simulink model "hdv_hydroelectropowertrain_model"  (R2023b)
settings: Solver=ode1be  StartTime=0.0  StopTime=simulation_length  FixedStep=tsample  MaxStep=tsample
values from neighbouring files (symbols this model uses):
  alpha = 35    [init_model.m]
  Apump = [0 1; 0 0]    [init_model.m]
  available_torque = torque_base+torque_friction_base    [init_model.m]
  Bpump = [0 1]'    [init_model.m]
  btheta_shaft = 2e2    (= 200)    [init_model.m]
  C1 = 10    [init_model.m]
  consumption = [consumption_1, consumption_2, consumption_3, consumption_4,          consumption_5, consumption_6, consumption_7, consumption_8,          consumption_9, consumption_10, consumption_11, consumption_12,          consumption_13, consumption_14, consumption_15, consumption_16          ]    [ic_engine_data.m]
  Cpump = [k 0]    [init_model.m]
  dp_lim = 400    [init_model.m]
  E0 = 3.685    [init_model.m]
  E1 = 0.2156    [init_model.m]
  E2 = 0    [init_model.m]
  E3 = 0    [init_model.m]
  E_1 = -1.031    [init_model.m]
  Elog = -0.05    [init_model.m]
  eta_v_m = 0.98    [init_model.m]
  eta_v_p = 0.97    [init_model.m]
  ki_dp_comp = 1/dp_lim    (= 0.0025)    [init_model.m]
  ki_te_comp = 2/te_lim    [init_model.m]
  kp_ctrl_m = 1    [init_model.m]
  kp_dp_comp = 0.5/dp_lim    (= 0.00125)    [init_model.m]
  kp_te_comp = 1/te_lim    [init_model.m]
  Kpump = acker(Apump,Bpump,poles)    [init_model.m]
  load_blade_enable = 0    [init_model.m]
  Lpump = acker(Apump',Cpump',pole_so)'    [init_model.m]
  M = 125    [init_model.m]
  Ncell = 185    [init_model.m]
  Npump = -1/(Cpump*inv(Apump-Bpump*Kpump)*Bpump)    [init_model.m]
  omega_e_rpm_ref = 1700    [init_model.m]
  omega_l_max_rpm = omega_l_max/(2*pi)*60    (= 50.3075969543)    [init_model.m]
  q1Kalman = tsample^2*1e-2    (= 1e-08)    [init_model.m]
  q2Kalman = tsample^1*1e-1    (= 0.0001)    [init_model.m]
  q3Kalman = 0    [init_model.m]
  Qhr = 400    [init_model.m]
  R0 = 0.015    [init_model.m]
  R1 = 0.015    [init_model.m]
  R_tg = 1.16/2    (= 0.58)    [init_model.m]
  rKalman = 1    [init_model.m]
  rpm_base = [620 700 800 900 1000 1100 1200 1300 1400 1500 1600 1700 1800      1900 2000 2100]    [ic_engine_data.m]
  rpm_consumption = rpm_base    [ic_engine_data.m]
  simulation_length = 245    [init_model.m]
  tau_load = 75e3    (= 75000)    [init_model.m]
  tau_load_max = 1600*41.4    (= 66240)    [init_model.m]
  Tc = tsample    (= 0.001)    [init_model.m]
  torque_base = [max(torque_16_data) max(torque_15_data) max(torque_14_data)      max(torque_13_data) max(torque_12_data) max(torque_11_data)      max(torque_10_data) max(torque_9_data) max(torque_8_data)      max(torque_7_data) max(torque_6_data) max(torque_5_data)      max(torque_4_data) max(torque_3_data) max(torque_2_data)      max(torque_1_data)]    [ic_engine_data.m]
  torque_consumption = torque_reference    [ic_engine_data.m]
  torque_friction_base = -(rpm_base./60*2*pi)*0.25-(rpm_base./60*2*pi).^2*5.2e-4    [ic_engine_data.m]
  tsample = 1e-3    (= 0.001)    [init_model.m]
  v_track1_ref = 8    [init_model.m]
  v_track2_ref = 8    [init_model.m]
  valve_mmorifice_max = 2.75    [init_model.m]
  xv_m_max = 1.2    [init_model.m]
undefined symbols (not defined in the file or in its folder): magnitude
libraries: fl_lib x381, nesl_utility x162, linear_swashplate_ctrl_lib x8, flexshaft_lib x5, bichamber_piston_lib x5, variable_displacement_motor_lib x4, variable_displacement_pump_lib x4, fixed_displacement_pump_lib x4, relief_valve_lib x4, inverse_shuttle_valve_lib x4, hydrostatic_threeway_valve_bichamber_piston_lib x4, hydrostatic_fourway_valve_bichamber_piston_lib x4
(part 1 of 9)
settings Model: SimulationMode=accelerator  Creator=dbagn  LastModifiedBy=dbagn
settings SolverCC: NumberNewtonIterations=3  AlgebraicLoopSolver=TrustRegion
settings DataIOCC: ReturnWorkspaceOutputs=off
settings DebuggingCC: UnconnectedInputMsg=warning  UnconnectedOutputMsg=warning  UnconnectedLineMsg=warning
settings ModelReferenceCC: EnableRefExpFcnMdlSchedulingChecks=on
settings RTWCC: DLArmComputeVersion=19.05

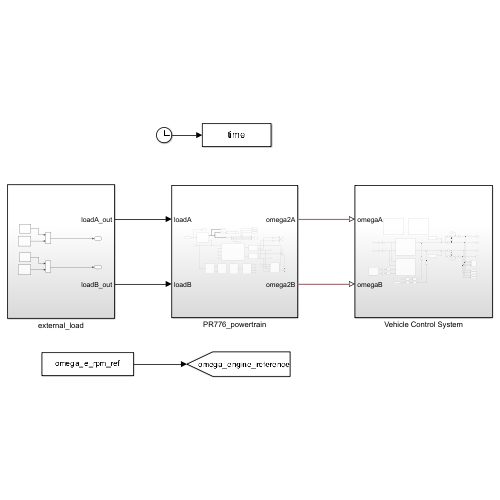
[thumbnail: Simulink's stored preview of the top-level diagram]
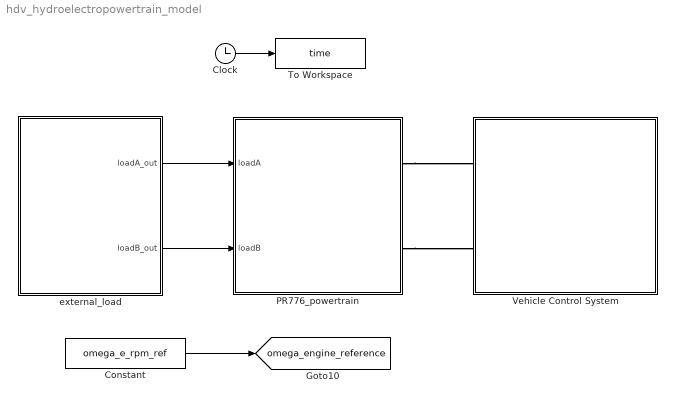
== system hdv_hydroelectropowertrain_model ==
  Clock : Clock
  Constant : Constant  Value=omega_e_rpm_ref
  PR776_powertrain : Subsystem
  To Workspace : ToWorkspace  VariableName=time  SampleTime=Tc
      settings: MaxDataPoints=Nc
  Vehicle Control System : Subsystem
  external_load : Subsystem
  tag scope: omega_engine_reference=global
  wires:
  Clock/1 -> To Workspace/1
  Constant/1 -> [omega_engine_reference]
  external_load/2(loadB_out) -> PR776_powertrain/2(loadB)
  external_load/1(loadA_out) -> PR776_powertrain/1(loadA)
  connections:
  PR776_powertrain/RConn1 -- Vehicle Control System/LConn1
  PR776_powertrain/RConn2 -- Vehicle Control System/LConn2

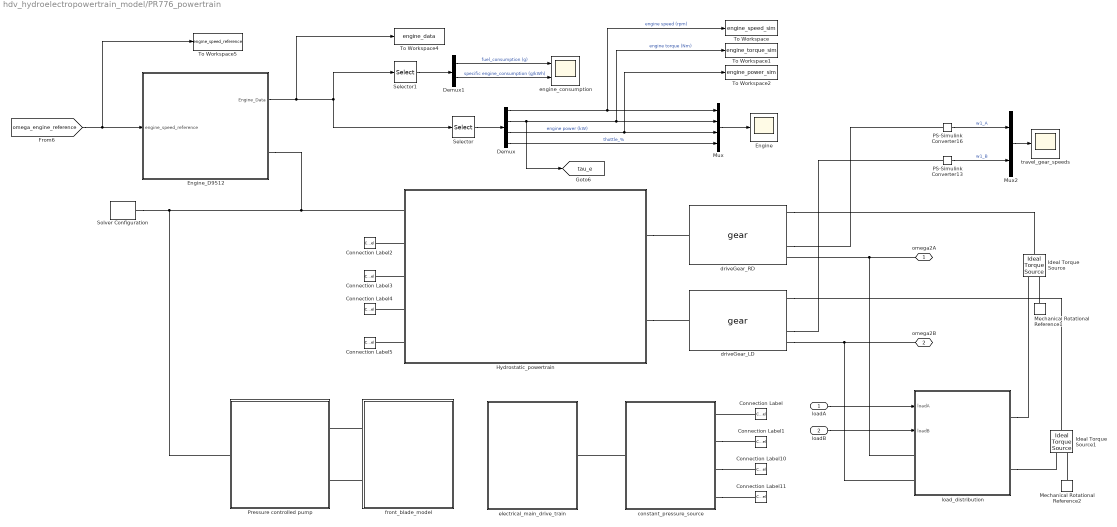
== system hdv_hydroelectropowertrain_model/PR776_powertrain ==
  loadA : Inport
  loadB : Inport  Port=2
  Connection Label : ConnectionLabel  Label=pS1
  Connection Label1 : ConnectionLabel  Label=pT1
  Connection Label10 : ConnectionLabel  Label=pS2
  Connection Label11 : ConnectionLabel  Label=pT2
  Connection Label2 : ConnectionLabel  Label=pS1
  Connection Label3 : ConnectionLabel  Label=pT1
  Connection Label4 : ConnectionLabel  Label=pS2
  Connection Label5 : ConnectionLabel  Label=pT2
  Demux : Demux
  Demux1 : Demux  Outputs=2
  Engine : Scope
  Engine_D9512 : Subsystem  mask(Internal Combustion Engine (ICE)){inertia=7.5, inertia_unit=kg*m^2, init_speed=5, diesel_density=0.85, diesel_density_unit=kg/l, rpm_base=rpm_base, rpm_base_unit=rpm, torque_friction_base=torque_friction_base, torque_friction_base_unit=N*m, torque_base=torque_base, torque_base_unit=N*m, rpm_consumption=rpm_consumption, rpm_consumption_unit=rpm, torque_consumption=torque_consumption, torque_consumption_unit=N*m, consumption=consumption, consumption_unit=g/(kW*hr), kp=2.5e-3, ki=2.5e-2, kd=0}
      mask prompts: init_speed "Initial Speed (RPM)"; diesel_density "Diesel density"; rpm_base "Base Speed Breakpoints"; torque_friction_base "Base Torque Friction Breakpoints"; torque_base "Base Torque Breakpoints"; rpm_consumption "Speed consumption breakpoints"; torque_consumption "Torque consumption breakpoints"; consumption "Consumption map"
      mask help:
      | This component models a generic internal combustion engine, modelled by means of introducing its characteristic performance maps.
      | Maps of main engine performance and of consumption have to be introduced. The component is also provided with a speed controller in which the PID gains can be introduced.
      mask init:
      | engine = [gcb, '/Generic Internal Combustion Engine'];
      | ctrl = [gcb, '/Engine Speed Controller'];
      | 
      | % Engine Parameters
      | set_param([engine],'cshaft_inertia','inertia');
      | set_param([engine],'cshaft_inertia_unit',inertia_unit);
      | set_param([engine],'initial_speed','init_speed');
      | set_param([engine],'diesel_density','diesel_density');
      | set_param([engine],'diesel_density_unit',diesel_density_unit);
      | 
      | % Tables
      | set_param([engine],'rpm_base','rpm_base');
      | set_param([engine],'torque_friction_base', 'torque_friction_base');
      | set_param([engine],'torque_base','torque_base');
      | set_param([engine],'rpm_consumption','rpm_consumption');
      | set_param([engine],'torque_consumption','torque_consumption');
      | set_param([engine],'consumption','consumption');
      | 
      | set_param([engine],'rpm_base_unit',rpm_base_unit);
      | set_param([engine],'torque_friction_base_unit',torque_friction_base_unit);
      | set_param([engine],'torque_base_unit',torque_base_unit);
      | set_param([engine],'rpm_consumption_unit',rpm_consumption_unit);
      | set_param([engine],'torque_consumption_unit',torque_consumption_unit);
      | set_param([engine],'consumption_unit',consumption_unit);
      | 
      | % Speed control
      | set_param([ctrl],'kp','kp');
      | set_param([ctrl],'kint','ki');
      | set_param([ctrl],'kd','kd');
      mask Help: eval('open \documentation\liebherr_engine_D9512_model_description.pdf')
      mask TypeOptions inertia_unit: kg*m^2
      mask TypeOptions diesel_density_unit: kg/l
      mask TypeOptions rpm_base_unit: rpm
      mask TypeOptions torque_friction_base_unit: N*m
      mask TypeOptions torque_base_unit: N*m
      mask TypeOptions rpm_consumption_unit: rpm
      mask TypeOptions torque_consumption_unit: kW
      mask TypeOptions consumption_unit: g/(kW*hr)
      mask DialogControl EngineParameters Prompt: Engine Parameters
      mask DialogControl Container5 Prompt: Engine Main Behaviour
      mask DialogControl Container4 Prompt: Consumption Behaviour
      mask DialogControl ControlParameters Prompt: Control Parameters
      mask Display:
      | modelname = [gcb];
      | % image(imread('Complementary/Pics/ICE.jpg'));
      | 
      | % color('red')
      | % port_label('lconn',1,'wref');
      | color('green')
      | port_label('rconn',1,'D');
      | color('black')
      | port_label('output',1,'Data');
      | port_label('input',1,'Engine Speed Reference');
  Hydrostatic_powertrain : Subsystem
  Ideal Torque Source : fl_lib/Mechanical/Mechanical Sources/Ideal Torque Source
  Ideal Torque Source1 : fl_lib/Mechanical/Mechanical Sources/Ideal Torque Source
  Mechanical Rotational Reference1 : fl_lib/Mechanical/Rotational Elements/Mechanical Rotational Reference
  Mechanical Rotational Reference2 : fl_lib/Mechanical/Rotational Elements/Mechanical Rotational Reference
  Mux : Mux
  Mux2 : Mux  Inputs=2
  PS-Simulink Converter13 : nesl_utility/PS-Simulink Converter  PhysicalDomain=network_engine_domain  SubClassName=ps_output  LeftPortType=input  RightPortType=output  PseudoPeriodic=off  Frequencies=[]  VectorFormat=1-D array  Unit=rpm  AffineConversion=on
  PS-Simulink Converter16 : nesl_utility/PS-Simulink Converter  PhysicalDomain=network_engine_domain  SubClassName=ps_output  LeftPortType=input  RightPortType=output  PseudoPeriodic=off  Frequencies=[]  VectorFormat=1-D array  Unit=rpm  AffineConversion=on
  Pressure controlled pump : Subsystem
  Selector : Selector  InputPortWidth=6  IndexOptions=Index vector (dialog)  Indices=[2 3 1 6]  OutputSizes=1
  Selector1 : Selector  InputPortWidth=6  IndexOptions=Index vector (dialog)  Indices=[5 4]  OutputSizes=1
  Solver Configuration : nesl_utility/Solver Configuration  PhysicalDomain=network_engine_domain  SubClassName=solver  LeftPortType=input  RightPortType=generic  Tones=[]  Harmonics=[]  SimulateNoise=off  Profile=off  UseLocalSampling=off  EnableSwitchedLinearOptims=on  FrequencyDomain=off  UseCCode=off  RelTol=0.001  AbsTol=1e-06  MinStep=1e-09  ToWorkspace=off  RevertToSquareIcSolve=off  NumHomotopyIterations=100  PhasorMode=off  PhasorModeNumHarmonics=1  ConsistencySolver=NEWTON_FTOL  IndexReductionMethod=DerivativeReplacement  DoDC=off  ResidualTolerance=tsample  ConsistencyTolSource=GLOBAL  ConsistencyAbsTol=0.001  ConsistencyRelTol=0.001  ConsistencyTolFactor=0.001  UseLocalSolver=on  LocalSolverChoice=NE_BACKWARD_EULER_ADVANCER  ResolveIndetEquations=on  FunctionEvalNumThread=1  LocalSolverSampleTime=tsample  DoFixedCost=on  MaxNonlinIter=3  MaxModeIter=2  ComputeImpulses=off  ImpulseIterations=2  LinearAlgebra=auto  LinearAlgebraNumThread=0  EquationFormulation=NE_TIME_EF  DelaysMemoryBudget=1024  AutomaticFiltering=on  FilteringTimeConstant=tsample  PartitionStorageMethod=AS_NEEDED  PartitionMemoryBudget=1024  PartitionMethod=ROBUST  MultibodyUseLocalSolver=off  MultibodyLocalSolverChoice=ODE1  MultibodyLocalSolverSampleTime=0.001
  To Workspace : ToWorkspace  VariableName=engine_speed_sim  SampleTime=Tc
      settings: MaxDataPoints=Nc
  To Workspace1 : ToWorkspace  VariableName=engine_torque_sim  SampleTime=Tc
      settings: MaxDataPoints=Nc
  To Workspace2 : ToWorkspace  VariableName=engine_power_sim  SampleTime=Tc
      settings: MaxDataPoints=Nc
  To Workspace4 : ToWorkspace  VariableName=engine_data  SampleTime=Tc
      settings: MaxDataPoints=Nc
  To Workspace5 : ToWorkspace  VariableName=engine_speed_reference  SampleTime=Tc
      settings: MaxDataPoints=Nc
  constant_pressure_source : Subsystem
  driveGear_LD : gear_lib/gear  n1=n_tg  n2=1  b1=b1 %0.02 N*m/(rad/s)  J1=0.25 kg*m^2  b2=track_friction_2 N*m/(rad/s)  J2=2 kg*m^2  k_theta_1=k_theta N*m/rad  w_1_specify=off  w_1_priority=None  w_1=0 rad/s  w_1_nominal_specify=off  w_1_nominal_unit=rad/s  w_1_nominal_value=1  w_2_specify=off  w_2_priority=None  w_2=0 rad/s  w_2_nominal_specify=off  w_2_nominal_unit=rad/s  w_2_nominal_value=1  t_1_specify=off  t_1_priority=None  t_1=0 N*m  t_1_nominal_specify=off  t_1_nominal_unit=N*m  t_1_nominal_value=1  t_2_specify=off  t_2_priority=None  t_2=0 N*m  t_2_nominal_specify=off  t_2_nominal_unit=N*m  t_2_nominal_value=1  t_theta_1_specify=off  t_theta_1_priority=None  t_theta_1=0 N*m  t_theta_1_nominal_specify=off  t_theta_1_nominal_unit=N*m  t_theta_1_nominal_value=1  t_theta_2_specify=off  t_theta_2_priority=None  t_theta_2=0 N*m  t_theta_2_nominal_specify=off  t_theta_2_nominal_unit=N*m  t_theta_2_nominal_value=1
      settings: InternalSimscapePortConfiguration="{\"Bottom\":[],\"Left\":[{\"id\":\"S1\",\"label\":\"S1\",\"type\":\"foundation.mechanical.rotational.rotational\"}],\"Right\":[{\"id\":\"S2\",\"label\":\"S2\",\"type\":\"foundation.mechanical.rotational.rotational\"},{\"id\":\"tau_theta_1\",\"label\":\"tau_theta_1\",\"type\":\"output\"},{\"id\":\"tau_theta_2\",\"label\":\"tau_theta_2\",\"type\":\"output\"},{\"id\":\"w1\",\"label\":\"w1\",\"type\":\"output\"},{\"id\":\"w2\",\"label\":\"w2\",\"type\":\"output\"}],\"Top\":[]}"
  driveGear_RD : gear_lib/gear  n1=n_tg  n2=1  b1=b1 %0.02 N*m/(rad/s)  J1=0.25 kg*m^2  b2=track_friction_1 N*m/(rad/s)  J2=2 kg*m^2  k_theta_1=k_theta N*m/rad  w_1_specify=off  w_1_priority=None  w_1=0 rad/s  w_1_nominal_specify=off  w_1_nominal_unit=rad/s  w_1_nominal_value=1  w_2_specify=off  w_2_priority=None  w_2=0 rad/s  w_2_nominal_specify=off  w_2_nominal_unit=rad/s  w_2_nominal_value=1  t_1_specify=off  t_1_priority=None  t_1=0 N*m  t_1_nominal_specify=off  t_1_nominal_unit=N*m  t_1_nominal_value=1  t_2_specify=off  t_2_priority=None  t_2=0 N*m  t_2_nominal_specify=off  t_2_nominal_unit=N*m  t_2_nominal_value=1  t_theta_1_specify=off  t_theta_1_priority=None  t_theta_1=0 N*m  t_theta_1_nominal_specify=off  t_theta_1_nominal_unit=N*m  t_theta_1_nominal_value=1  t_theta_2_specify=off  t_theta_2_priority=None  t_theta_2=0 N*m  t_theta_2_nominal_specify=off  t_theta_2_nominal_unit=N*m  t_theta_2_nominal_value=1
      settings: InternalSimscapePortConfiguration="{\"Bottom\":[],\"Left\":[{\"id\":\"S1\",\"label\":\"S1\",\"type\":\"foundation.mechanical.rotational.rotational\"}],\"Right\":[{\"id\":\"S2\",\"label\":\"S2\",\"type\":\"foundation.mechanical.rotational.rotational\"},{\"id\":\"tau_theta_1\",\"label\":\"tau_theta_1\",\"type\":\"output\"},{\"id\":\"tau_theta_2\",\"label\":\"tau_theta_2\",\"type\":\"output\"},{\"id\":\"w1\",\"label\":\"w1\",\"type\":\"output\"},{\"id\":\"w2\",\"label\":\"w2\",\"type\":\"output\"}],\"Top\":[]}"
  electrical_main_drive_train : Subsystem
  engine_consumption : Scope  NumInputPorts=2
  front_blade_model : Subsystem
  load_distribution : Subsystem
  travel_gear_speeds : Scope
  omega2A : PMIOPort  Side=Right
  omega2B : PMIOPort  Port=2  Side=Right
  tag scope: tau_e=global
  wires:
  Demux/2 -> [tau_e], To Workspace1/1, Mux/2  "engine torque (Nm)"
  Demux/1 -> To Workspace/1, Mux/1  "engine speed (rpm)"
  Mux/1 -> Engine/1
  Demux/4 -> Mux/4  "thottle_%"
  Demux/3 -> Mux/3, To Workspace2/1  "engine power (kW)"
  PS-Simulink Converter13/1 -> Mux2/2  "w1_B"
  PS-Simulink Converter16/1 -> Mux2/1  "w1_A"
  Mux2/1 -> travel_gear_speeds/1
  loadA/1 -> load_distribution/1(loadA)
  loadB/1 -> load_distribution/2(loadB)
  Demux1/2 -> engine_consumption/2  "specific engine_consumption (g/kWh)"
  Demux1/1 -> engine_consumption/1  "fuel_consumption (g)"
  [omega_engine_reference] -> Engine_D9512/1(engine_speed_reference), To Workspace5/1
  Selector/1 -> Demux/1
  Selector1/1 -> Demux1/1
  Engine_D9512/1(Engine_Data) -> To Workspace4/1, Selector/1, Selector1/1
  connections:
  Mechanical Rotational Reference1/LConn1 -- Ideal Torque Source/RConn2
  driveGear_LD/RConn5 -- load_distribution/LConn2 -- omega2B/RConn1
  Mechanical Rotational Reference2/LConn1 -- Ideal Torque Source1/RConn2
  omega2A/RConn1 -- load_distribution/LConn1 -- driveGear_RD/RConn5
  driveGear_LD/RConn4 -- PS-Simulink Converter13/LConn1
  driveGear_RD/RConn4 -- PS-Simulink Converter16/LConn1
  driveGear_RD/RConn1 -- Ideal Torque Source/LConn1
  driveGear_LD/RConn1 -- Ideal Torque Source1/LConn1
  load_distribution/RConn1 -- Ideal Torque Source/RConn1
  load_distribution/RConn2 -- Ideal Torque Source1/RConn1
  Hydrostatic_powertrain/RConn1 -- driveGear_RD/LConn1
  Solver Configuration/RConn1 -- Pressure controlled pump/LConn1 -- Hydrostatic_powertrain/LConn1 -- Engine_D9512/RConn1
  Hydrostatic_powertrain/RConn2 -- driveGear_LD/LConn1
  Hydrostatic_powertrain/LConn2 -- Connection Label2/LConn1
  Hydrostatic_powertrain/LConn3 -- Connection Label3/LConn1
  Hydrostatic_powertrain/LConn5 -- Connection Label5/LConn1
  Hydrostatic_powertrain/LConn4 -- Connection Label4/LConn1
  front_blade_model/LConn2 -- Pressure controlled pump/RConn2
  front_blade_model/LConn1 -- Pressure controlled pump/RConn1
  constant_pressure_source/LConn1 -- electrical_main_drive_train/RConn1
  constant_pressure_source/RConn3 -- Connection Label10/LConn1
  constant_pressure_source/RConn4 -- Connection Label11/LConn1
  Connection Label/LConn1 -- constant_pressure_source/RConn1
  constant_pressure_source/RConn2 -- Connection Label1/LConn1

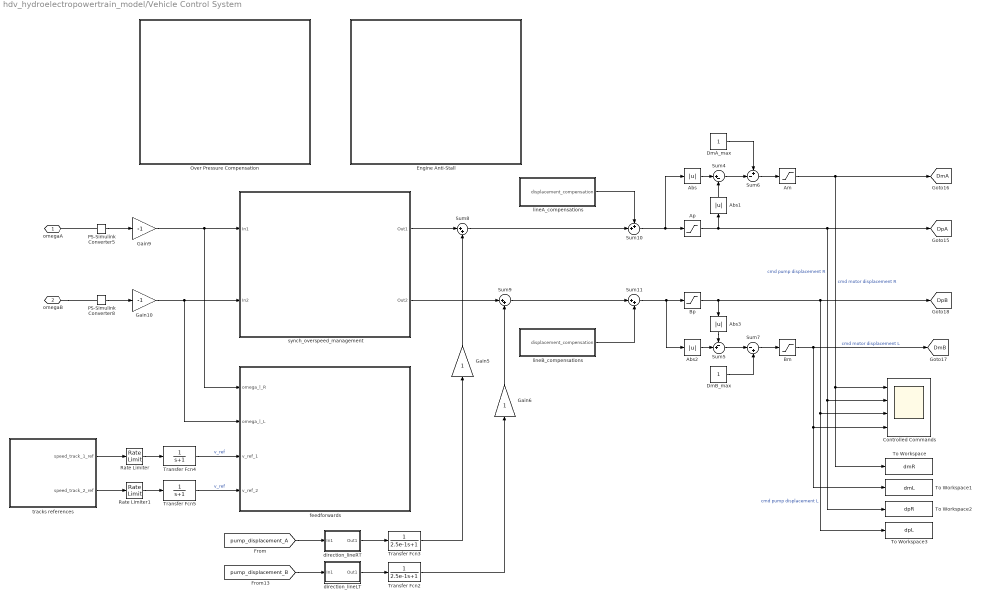
== system hdv_hydroelectropowertrain_model/Vehicle Control System ==
  Abs{,1..3} (4 alike) : Abs  SaturateOnIntegerOverflow=off
  Am : Saturate  UpperLimit=1  LowerLimit=0.36
  Ap : Saturate  UpperLimit=1  LowerLimit=-1
  Bm : Saturate  UpperLimit=1  LowerLimit=0.36
  Bp : Saturate  UpperLimit=1  LowerLimit=-1
  Controlled Commands : Scope  NumInputPorts=4
  DmA_max : Constant
  DmB_max : Constant
  Engine Anti-Stall : Subsystem
  Gain10 : Gain  Gain=-1
  Gain5 : Gain
  Gain6 : Gain
  Gain9 : Gain  Gain=-1
  Over Pressure Compensation : Subsystem
  PS-Simulink Converter5 : nesl_utility/PS-Simulink Converter  PhysicalDomain=network_engine_domain  SubClassName=ps_output  LeftPortType=input  RightPortType=output  PseudoPeriodic=off  Frequencies=[]  VectorFormat=1-D array  Unit=rpm  AffineConversion=off
  PS-Simulink Converter8 : nesl_utility/PS-Simulink Converter  PhysicalDomain=network_engine_domain  SubClassName=ps_output  LeftPortType=input  RightPortType=output  PseudoPeriodic=off  Frequencies=[]  VectorFormat=1-D array  Unit=rpm  AffineConversion=off
  Rate Limiter : RateLimiter  RisingSlewLimit=v_track1_ref/4  FallingSlewLimit=-v_track1_ref/4  SampleTimeMode=inherited
  Rate Limiter1 : RateLimiter  RisingSlewLimit=v_track2_ref/4  FallingSlewLimit=-v_track2_ref/4  SampleTimeMode=inherited
  Sum10 : Sum  Inputs=++|
  Sum11 : Sum  Inputs=|++
  Sum4 : Sum  Inputs=|+-
  Sum5 : Sum  Inputs=-+|
  Sum6 : Sum  Inputs=+-|
  Sum7 : Sum  Inputs=|-+
  Sum8 : Sum  Inputs=|++
  Sum9 : Sum  Inputs=|++
  To Workspace : ToWorkspace  VariableName=dmR  SampleTime=Tc
      settings: MaxDataPoints=Nc
  To Workspace1 : ToWorkspace  VariableName=dmL  SampleTime=Tc
      settings: MaxDataPoints=Nc
  To Workspace2 : ToWorkspace  VariableName=dpR  SampleTime=Tc
      settings: MaxDataPoints=Nc
  To Workspace3 : ToWorkspace  VariableName=dpL  SampleTime=Tc
      settings: MaxDataPoints=Nc
  Transfer Fcn2 : TransferFcn  Denominator=[2.5e-1 1]
  Transfer Fcn3 : TransferFcn  Denominator=[2.5e-1 1]
  Transfer Fcn4 : TransferFcn  Denominator=[1 1]
  Transfer Fcn5 : TransferFcn  Denominator=[1 1]
  direction_lineLT : Subsystem
  direction_lineRT : Subsystem
  feedforwards : Subsystem
  lineA_compensations : Subsystem
  "lineB_compensations " : Subsystem
  synch_overspeed_management : Subsystem
  tracks references : Subsystem
  omegaA : PMIOPort  Side=Left
  omegaB : PMIOPort  Port=2  Side=Left
  tag scope: DmA=global, DmB=global, DpA=global, DpB=global
  wires:
  Sum4/1 -> Sum6/2
  DmA_max/1 -> Sum6/1
  Sum6/1 -> Am/1
  DmB_max/1 -> Sum7/2
  Sum5/1 -> Sum7/1
  Sum7/1 -> Bm/1
  [pump_displacement_B] -> direction_lineLT/1(In1)
  [pump_displacement_A] -> direction_lineRT/1(In1)
  Abs/1 -> Sum4/1
  Abs1/1 -> Sum4/2
  Abs2/1 -> Sum5/2
  Abs3/1 -> Sum5/1
  Sum8/1 -> Sum10/2
  Sum9/1 -> Sum11/1
  Sum10/1 -> Abs/1, Ap/1
  Sum11/1 -> Bp/1, Abs2/1
  lineA_compensations/1(displacement_compensation) -> Sum10/1
  "lineB_compensations "/1(displacement_compensation) -> Sum11/2
  Bp/1 -> [DpB], To Workspace3/1, Controlled Commands/3, Abs3/1  "cmd pump displacement L"
  Ap/1 -> [DpA], To Workspace2/1, Controlled Commands/2, Abs1/1  "cmd pump displacement R"
  Am/1 -> [DmA], To Workspace/1, Controlled Commands/1  "cmd motor displacement R"
  Bm/1 -> [DmB], Controlled Commands/4, To Workspace1/1  "cmd motor displacement L"
  Transfer Fcn3/1 -> Gain5/1
  Transfer Fcn2/1 -> Gain6/1
  direction_lineRT/1(Out1) -> Transfer Fcn3/1
  direction_lineLT/1(Out1) -> Transfer Fcn2/1
  Gain5/1 -> Sum8/2
  Gain6/1 -> Sum9/2
  Gain10/1 -> feedforwards/2(omega_l_L), synch_overspeed_management/2(In2)
  Gain9/1 -> feedforwards/1(omega_l_R), synch_overspeed_management/1(In1)
  PS-Simulink Converter8/1 -> Gain10/1
  PS-Simulink Converter5/1 -> Gain9/1
  Rate Limiter/1 -> Transfer Fcn4/1
  Rate Limiter1/1 -> Transfer Fcn5/1
  Transfer Fcn4/1 -> feedforwards/3(v_ref_1)  "v_ref"
  Transfer Fcn5/1 -> feedforwards/4(v_ref_2)  "v_ref"
  synch_overspeed_management/1(Out1) -> Sum8/1
  synch_overspeed_management/2(Out2) -> Sum9/1
  tracks references/1(speed_track_1_ref) -> Rate Limiter/1
  tracks references/2(speed_track_2_ref) -> Rate Limiter1/1
  connections:
  omegaB/RConn1 -- PS-Simulink Converter8/LConn1
  PS-Simulink Converter5/LConn1 -- omegaA/RConn1

== system hdv_hydroelectropowertrain_model/external_load ==
  Product1 : Product
  Product3 : Product
  Q1 : Constant  Value=-1
  Q2 : Constant  Value=-1
  loadA : Subsystem
  loadB : Subsystem
  loadA_out : Outport
  loadB_out : Outport  Port=2
  wires:
  loadB/1(Out1) -> Product3/2
  loadA/1(Out1) -> Product1/2
  Q2/1 -> Product3/1
  Q1/1 -> Product1/1
  Product1/1 -> loadA_out/1
  Product3/1 -> loadB_out/1

== system hdv_hydroelectropowertrain_model/PR776_powertrain/Engine_D9512 ==
  engine_speed_reference : Inport
  Bus Creator : BusCreator  Inputs=6
  Engine Speed Controller : engine_speed_ctrl_ii_lib/Engine Speed Controller UD  kp=kp s  kint=ki  kd=kd s^2  t_out_specify=off  t_out_priority=None  t_out=0.0  t_out_nominal_specify=off  t_out_nominal_unit=1  t_out_nominal_value=1
      settings: InternalSimscapePortConfiguration="{\"Bottom\":[],\"Left\":[{\"id\":\"we_ref\",\"label\":\"we_ref\",\"type\":\"input\"},{\"id\":\"we\",\"label\":\"we\",\"type\":\"input\"}],\"Right\":[{\"id\":\"theta\",\"label\":\"tS\",\"type\":\"output\"}],\"Top\":[]}"
  Generic Internal Combustion Engine : ice_lib/Generic Internal Combustion Engine  cshaft_inertia=inertia kg*m^2  initial_speed=init_speed  diesel_density=diesel_density kg/l  rpm_consumption=rpm_consumption rpm  torque_consumption=torque_consumption N*m  consumption=consumption g/(kW*hr)  rpm_base=rpm_base rpm  torque_friction_base=torque_friction_base N*m  torque_base=torque_base N*m
      settings: InternalSimscapePortConfiguration="{\"Bottom\":[],\"Left\":[{\"id\":\"theta\",\"label\":\"theta\",\"type\":\"input\"},{\"id\":\"C\",\"label\":\"C\",\"type\":\"foundation.mechanical.rotational.rotational\"}],\"Right\":[{\"id\":\"Pe\",\"label\":\"Pe\",\"type\":\"output\"},{\"id\":\"omega_e_out\",\"label\":\"omega_e\",\"type\":\"output\"},{\"id\":\"tau_d_out\",\"label\":\"tau_d\",\"type\":\"output\"},{\"id\":\"sfc\",\"label\":\"sfc\",\"type\":\"output\"},{\"id\":\"fc\",\"label\":\"fc\",\"type\":\"output\"},{\"id\":\"D\",\"label\":\"D\",\"type\":\"foundation.mechanical.rotational.rotational\"}],\"Top\":[]}"
  Mechanical Rotational Reference : fl_lib/Mechanical/Rotational Elements/Mechanical Rotational Reference
  PS-Simulink Converter1 : nesl_utility/PS-Simulink Converter  PhysicalDomain=network_engine_domain  SubClassName=ps_output  LeftPortType=input  RightPortType=output  PseudoPeriodic=off  Frequencies=[]  VectorFormat=1-D array  Unit=N*m  AffineConversion=on
  PS-Simulink Converter2 : nesl_utility/PS-Simulink Converter  PhysicalDomain=network_engine_domain  SubClassName=ps_output  LeftPortType=input  RightPortType=output  PseudoPeriodic=off  Frequencies=[]  VectorFormat=1-D array  Unit=rpm  AffineConversion=on
  PS-Simulink Converter5 : nesl_utility/PS-Simulink Converter  PhysicalDomain=network_engine_domain  SubClassName=ps_output  LeftPortType=input  RightPortType=output  PseudoPeriodic=off  Frequencies=[]  VectorFormat=1-D array  Unit=g/(kW*hr)  AffineConversion=on
  PS-Simulink Converter6 : nesl_utility/PS-Simulink Converter  PhysicalDomain=network_engine_domain  SubClassName=ps_output  LeftPortType=input  RightPortType=output  PseudoPeriodic=off  Frequencies=[]  VectorFormat=1-D array  Unit=kW  AffineConversion=on
  PS-Simulink Converter7 : nesl_utility/PS-Simulink Converter  PhysicalDomain=network_engine_domain  SubClassName=ps_output  LeftPortType=input  RightPortType=output  PseudoPeriodic=off  Frequencies=[]  VectorFormat=1-D array  Unit=l  AffineConversion=on
  PS-Simulink Converter8 : nesl_utility/PS-Simulink Converter  PhysicalDomain=network_engine_domain  SubClassName=ps_output  LeftPortType=input  RightPortType=output  PseudoPeriodic=off  Frequencies=[]  VectorFormat=1-D array  Unit=1  AffineConversion=on
  Simulink-PS Converter7 : nesl_utility/Simulink-PS Converter  PhysicalDomain=network_engine_domain  SubClassName=ps_input  LeftPortType=input  RightPortType=output  PseudoPeriodic=off  Frequencies=[]  NoiseDistribution=none  NoiseParameters=[]  Unit=rpm  AffineConversion=on  FilteringAndDerivatives=provide  SimscapeFilterOrder=1  InputFilterTimeConstant=0.001  UdotUserProvided=0
  D : PMIOPort  Side=Right
  Engine_Data : Outport
  wires:
  PS-Simulink Converter2/1 -> Bus Creator/2  "engine speed (rpm)"
  PS-Simulink Converter5/1 -> Bus Creator/4  "engine specific consumption (g/kWh)"
  PS-Simulink Converter1/1 -> Bus Creator/3  "engine available torque (N*m)"
  Bus Creator/1 -> Engine_Data/1
  PS-Simulink Converter7/1 -> Bus Creator/5  "engine consumption (l)"
  PS-Simulink Converter6/1 -> Bus Creator/1  "engine power (consumption) (kW)"
  PS-Simulink Converter8/1 -> Bus Creator/6  "throttle"
  engine_speed_reference/1 -> Simulink-PS Converter7/1
  connections:
  Generic Internal Combustion Engine/LConn2 -- Mechanical Rotational Reference/LConn1
  Generic Internal Combustion Engine/RConn1 -- PS-Simulink Converter6/LConn1
  Generic Internal Combustion Engine/RConn6 -- D/RConn1
  PS-Simulink Converter2/LConn1 -- Generic Internal Combustion Engine/RConn2 -- Engine Speed Controller/LConn2
  Generic Internal Combustion Engine/RConn4 -- PS-Simulink Converter5/LConn1
  Generic Internal Combustion Engine/RConn3 -- PS-Simulink Converter1/LConn1
  PS-Simulink Converter8/LConn1 -- Engine Speed Controller/RConn1 -- Generic Internal Combustion Engine/LConn1
  Generic Internal Combustion Engine/RConn5 -- PS-Simulink Converter7/LConn1
  Engine Speed Controller/LConn1 -- Simulink-PS Converter7/RConn1

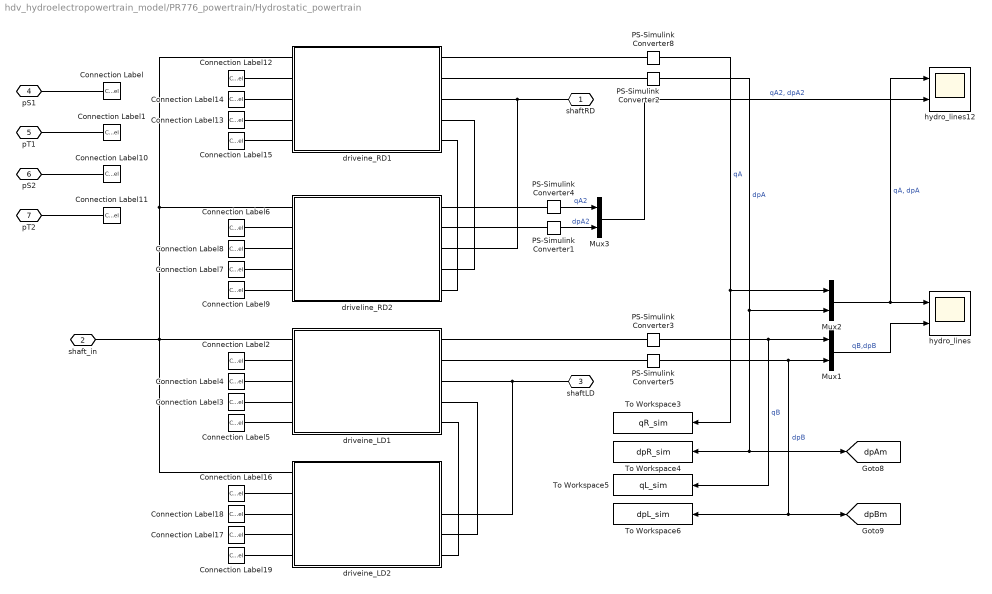
== system hdv_hydroelectropowertrain_model/PR776_powertrain/Hydrostatic_powertrain ==
  Connection Label{,2,6,12,16} (5 alike) : ConnectionLabel  Label=pS1
  Connection Label{1,3,7,13,17} (5 alike) : ConnectionLabel  Label=pT1
  Connection Label{4,8,10,14,18} (5 alike) : ConnectionLabel  Label=pS2
  Connection Label{5,9,11,15,19} (5 alike) : ConnectionLabel  Label=pT2
  Mux1 : Mux  Inputs=2
  Mux2 : Mux  Inputs=2
  Mux3 : Mux  Inputs=2
  PS-Simulink Converter1 : nesl_utility/PS-Simulink Converter  PhysicalDomain=network_engine_domain  SubClassName=ps_output  LeftPortType=input  RightPortType=output  PseudoPeriodic=off  Frequencies=[]  VectorFormat=1-D array  Unit=bar  AffineConversion=off
  PS-Simulink Converter2 : nesl_utility/PS-Simulink Converter  PhysicalDomain=network_engine_domain  SubClassName=ps_output  LeftPortType=input  RightPortType=output  PseudoPeriodic=off  Frequencies=[]  VectorFormat=1-D array  Unit=bar  AffineConversion=off
  PS-Simulink Converter3 : nesl_utility/PS-Simulink Converter  PhysicalDomain=network_engine_domain  SubClassName=ps_output  LeftPortType=input  RightPortType=output  PseudoPeriodic=off  Frequencies=[]  VectorFormat=1-D array  Unit=l/min  AffineConversion=off
  PS-Simulink Converter4 : nesl_utility/PS-Simulink Converter  PhysicalDomain=network_engine_domain  SubClassName=ps_output  LeftPortType=input  RightPortType=output  PseudoPeriodic=off  Frequencies=[]  VectorFormat=1-D array  Unit=l/min  AffineConversion=off
  PS-Simulink Converter5 : nesl_utility/PS-Simulink Converter  PhysicalDomain=network_engine_domain  SubClassName=ps_output  LeftPortType=input  RightPortType=output  PseudoPeriodic=off  Frequencies=[]  VectorFormat=1-D array  Unit=bar  AffineConversion=off
  PS-Simulink Converter8 : nesl_utility/PS-Simulink Converter  PhysicalDomain=network_engine_domain  SubClassName=ps_output  LeftPortType=input  RightPortType=output  PseudoPeriodic=off  Frequencies=[]  VectorFormat=1-D array  Unit=l/min  AffineConversion=off
  To Workspace3 : ToWorkspace  VariableName=qR_sim  SampleTime=Tc
      settings: MaxDataPoints=Nc
  To Workspace4 : ToWorkspace  VariableName=dpR_sim  SampleTime=Tc
      settings: MaxDataPoints=Nc
  To Workspace5 : ToWorkspace  VariableName=qL_sim  SampleTime=Tc
      settings: MaxDataPoints=Nc
  To Workspace6 : ToWorkspace  VariableName=dpL_sim  SampleTime=Tc
      settings: MaxDataPoints=Nc
  driveine_LD1 : Subsystem
  driveine_LD2 : Subsystem
  driveine_RD1 : Subsystem
  driveline_RD2 : Subsystem
  hydro_lines : Scope  NumInputPorts=2
  hydro_lines12 : Scope  NumInputPorts=2
  shaftRD : PMIOPort  Side=Right
  shaft_in : PMIOPort  Port=2  Side=Left
  shaftLD : PMIOPort  Port=3  Side=Right
  pS1 : PMIOPort  Port=4  Side=Left
  pT1 : PMIOPort  Port=5  Side=Left
  pS2 : PMIOPort  Port=6  Side=Left
  pT2 : PMIOPort  Port=7  Side=Left
  tag scope: dpAm=global, dpBm=global
  wires:
  PS-Simulink Converter2/1 -> [dpAm], To Workspace4/1, Mux2/2  "dpA"
  PS-Simulink Converter3/1 -> Mux1/1, To Workspace5/1  "qB"
  PS-Simulink Converter8/1 -> Mux2/1, To Workspace3/1  "qA"
  PS-Simulink Converter5/1 -> [dpBm], To Workspace6/1, Mux1/2  "dpB"
  Mux2/1 -> hydro_lines12/1, hydro_lines/1  "qA, dpA"
  Mux1/1 -> hydro_lines/2  "qB,dpB"
  PS-Simulink Converter4/1 -> Mux3/1  "qA2"
  PS-Simulink Converter1/1 -> Mux3/2  "dpA2"
  Mux3/1 -> hydro_lines12/2  "qA2, dpA2"
  connections:
  shaft_in/RConn1 -- driveine_RD1/LConn1 -- driveline_RD2/LConn1 -- driveine_LD2/LConn1 -- driveine_LD1/LConn1
  pT1/RConn1 -- Connection Label1/LConn1
  pS1/RConn1 -- Connection Label/LConn1
  pS2/RConn1 -- Connection Label10/LConn1
  pT2/RConn1 -- Connection Label11/LConn1
  driveine_RD1/RConn1 -- PS-Simulink Converter8/LConn1
  driveine_RD1/RConn2 -- PS-Simulink Converter2/LConn1
  driveine_RD1/RConn3 -- driveline_RD2/RConn3 -- shaftRD/RConn1
  Connection Label9/LConn1 -- driveline_RD2/LConn5
  Connection Label7/LConn1 -- driveline_RD2/LConn4
  Connection Label8/LConn1 -- driveline_RD2/LConn3
  Connection Label6/LConn1 -- driveline_RD2/LConn2
  Connection Label15/LConn1 -- driveine_RD1/LConn5
  Connection Label13/LConn1 -- driveine_RD1/LConn4
  Connection Label14/LConn1 -- driveine_RD1/LConn3
  Connection Label12/LConn1 -- driveine_RD1/LConn2
  driveine_LD1/RConn3 -- driveine_LD2/RConn3 -- shaftLD/RConn1
  Connection Label2/LConn1 -- driveine_LD1/LConn2
  Connection Label4/LConn1 -- driveine_LD1/LConn3
  Connection Label3/LConn1 -- driveine_LD1/LConn4
  Connection Label5/LConn1 -- driveine_LD1/LConn5
  Connection Label16/LConn1 -- driveine_LD2/LConn2
  Connection Label18/LConn1 -- driveine_LD2/LConn3
  Connection Label17/LConn1 -- driveine_LD2/LConn4
  Connection Label19/LConn1 -- driveine_LD2/LConn5
  driveine_RD1/RConn4 -- driveline_RD2/RConn4
  driveine_RD1/RConn5 -- driveline_RD2/RConn5
  driveine_LD1/RConn4 -- driveine_LD2/RConn4
  driveine_LD1/RConn5 -- driveine_LD2/RConn5
  driveine_LD1/RConn1 -- PS-Simulink Converter3/LConn1
  driveine_LD1/RConn2 -- PS-Simulink Converter5/LConn1
  driveline_RD2/RConn2 -- PS-Simulink Converter1/LConn1
  PS-Simulink Converter4/LConn1 -- driveline_RD2/RConn1

== system hdv_hydroelectropowertrain_model/PR776_powertrain/Pressure controlled pump ==
  Hydraulic Flow Rate Sensor : fl_lib/Hydraulic/Hydraulic Sensors/Hydraulic Flow Rate Sensor
  Hydraulic Pressure Sensor : fl_lib/Hydraulic/Hydraulic Sensors/Hydraulic Pressure Sensor
  Hydraulic Reference : fl_lib/Hydraulic/Hydraulic Elements/Hydraulic Reference
  PS Step : fl_lib/Physical Signals/Sources/PS Step  step_time=20 s  initial_value=32 bar  final_value=250 bar
  PS-Simulink Converter : nesl_utility/PS-Simulink Converter  PhysicalDomain=network_engine_domain  SubClassName=ps_output  LeftPortType=input  RightPortType=output  PseudoPeriodic=off  Frequencies=[]  VectorFormat=1-D array  Unit=bar  AffineConversion=on
  PS-Simulink Converter1 : nesl_utility/PS-Simulink Converter  PhysicalDomain=network_engine_domain  SubClassName=ps_output  LeftPortType=input  RightPortType=output  PseudoPeriodic=off  Frequencies=[]  VectorFormat=1-D array  Unit=l/min  AffineConversion=on
  PS-Simulink Converter{2..5} (4 alike) : nesl_utility/PS-Simulink Converter  PhysicalDomain=network_engine_domain  SubClassName=ps_output  LeftPortType=input  RightPortType=output  PseudoPeriodic=off  Frequencies=[]  VectorFormat=1-D array  Unit=1  AffineConversion=off
  Pressure controlled pump : pressure_controlled_pump_lib/Pressure controlled pump  Vd_nom=90 %62.3 cm^3/rev  pnom=250 bar  b=0.124 N*m/(rad/s)  inertia_pump=0.027 kg*m^2  vd_lim_max=0.98  vd_lim_min=0  p_set=258 bar  p_reg=12 bar  x_rv_max=10 mm  kpc=8  kic=8 1/s  te_specify=off  te_priority=None  te=0 N*m  te_nominal_specify=off  te_nominal_unit=N*m  te_nominal_value=1  qA_specify=off  qA_priority=None  qA=0 m^3/s  qA_nominal_specify=off  qA_nominal_unit=m^3/s  qA_nominal_value=1  qB_specify=off  qB_priority=None  qB=0 m^3/s  qB_nominal_specify=off  qB_nominal_unit=m^3/s  qB_nominal_value=1  qd_specify=off  qd_priority=None  qd=0 m^3/s  qd_nominal_specify=off  qd_nominal_unit=m^3/s  qd_nominal_value=1  dp_specify=off  dp_priority=None  dp=0 Pa  dp_nominal_specify=off  dp_nominal_unit=Pa  dp_nominal_value=1  vd_specify=off  vd_priority=None  vd=0  vd_nominal_specify=off  vd_nominal_unit=1  vd_nominal_value=1  vd_i_specify=off  vd_i_priority=None  vd_i=0  vd_i_nominal_specify=off  vd_i_nominal_unit=1  vd_i_nominal_value=1  we_specify=off  we_priority=None  we=0 rad/s  we_nominal_specify=off  we_nominal_unit=rad/s  we_nominal_value=1
      settings: InternalSimscapePortConfiguration="{\"Bottom\":[],\"Left\":[{\"id\":\"cW\",\"label\":\"cW\",\"type\":\"foundation.mechanical.rotational.rotational\"},{\"id\":\"dp_ref\",\"label\":\"Pressure set-point\",\"type\":\"input\"}],\"Right\":[{\"id\":\"cA\",\"label\":\"cA\",\"type\":\"foundation.hydraulic.hydraulic\"},{\"id\":\"cB\",\"label\":\"cB\",\"type\":\"foundation.hydraulic.hydraulic\"},{\"id\":\"qleak\",\"label\":\"qleak\",\"type\":\"output\"},{\"id\":\"taup\",\"label\":\"taup\",\"type\":\"output\"},{\"id\":\"vdi\",\"label\":\"vdi\",\"type\":\"output\"},{\"id\":\"pflow\",\"label\":\"pflow\",\"type\":\"output\"}],\"Top\":[]}"
  flow : Scope
  leak/ptorque : Scope  NumInputPorts=3
  pressure : Scope
  pump_flow : Scope
  pS : PMIOPort  Side=Right
  shaft : PMIOPort  Port=2  Side=Left
  pT : PMIOPort  Port=3  Side=Right
  wires:
  PS-Simulink Converter1/1 -> flow/1
  PS-Simulink Converter4/1 -> leak/ptorque/3  "vd"
  PS-Simulink Converter3/1 -> leak/ptorque/2  "torque"
  PS-Simulink Converter5/1 -> pump_flow/1
  PS-Simulink Converter2/1 -> leak/ptorque/1  "leak"
  PS-Simulink Converter/1 -> pressure/1
  connections:
  shaft/RConn1 -- Pressure controlled pump/LConn1
  Pressure controlled pump/RConn4 -- PS-Simulink Converter3/LConn1
  Pressure controlled pump/RConn3 -- PS-Simulink Converter2/LConn1
  Hydraulic Flow Rate Sensor/RConn1 -- PS-Simulink Converter1/LConn1
  Hydraulic Pressure Sensor/LConn1 -- pS/RConn1 -- Hydraulic Flow Rate Sensor/RConn2
  Hydraulic Reference/LConn1 -- Pressure controlled pump/RConn2 -- pT/RConn1 -- Hydraulic Pressure Sensor/RConn1
  Pressure controlled pump/RConn1 -- Hydraulic Flow Rate Sensor/LConn1
  Pressure controlled pump/RConn5 -- PS-Simulink Converter4/LConn1
  Pressure controlled pump/RConn6 -- PS-Simulink Converter5/LConn1
  PS-Simulink Converter/LConn1 -- Hydraulic Pressure Sensor/RConn2
  PS Step/RConn1 -- Pressure controlled pump/LConn2

== system hdv_hydroelectropowertrain_model/PR776_powertrain/constant_pressure_source ==
  Pressure controlled pump : Subsystem
  Pressure controlled pump1 : Subsystem
  pS1 : PMIOPort  Side=Right
  pT1 : PMIOPort  Port=2  Side=Right
  pS2 : PMIOPort  Port=3  Side=Right
  pT2 : PMIOPort  Port=4  Side=Right
  C : PMIOPort  Port=5  Side=Left
  connections:
  Pressure controlled pump/RConn1 -- pS1/RConn1
  Pressure controlled pump/RConn2 -- pT1/RConn1
  Pressure controlled pump1/LConn1 -- Pressure controlled pump/LConn1 -- C/RConn1
  Pressure controlled pump1/RConn2 -- pT2/RConn1
  Pressure controlled pump1/RConn1 -- pS2/RConn1

== system hdv_hydroelectropowertrain_model/PR776_powertrain/electrical_main_drive_train ==
  DCDC_Data : Scope
  Demux : Demux  Outputs=2
  LithiumIonBattery : Subsystem  mask{Q=Qhr, Q_unit=A*hr, Ncell=Ncell, E_1=E_1, E_1_unit=V, E0=E0, E0_unit=V, E1=E1, E1_unit=V, E2=E2, E2_unit=V, E3=E3, E3_unit=V, Elog=Elog, Elog_unit=V, R0=R0, R0_unit=Ohm, R1=R1, R1_unit=Ohm, C1=C1, C1_unit=F, M=M, M_unit=V, alpha=alpha}
      mask prompts: Q "Charge Capacity"; Ncell "Number of Cells"
      mask init:
      | LithiumIonBattery = [gcb, '/lithium ion cell analytical ocv/lithium-ion battery with analytical OCV'];
      | set_param([LithiumIonBattery],'Qcell','Q');
      | set_param([LithiumIonBattery],'Qcell_unit',Q_unit);
      | set_param([LithiumIonBattery],'N','Ncell');
      | set_param([LithiumIonBattery],'E_1','E_1');
      | set_param([LithiumIonBattery],'E_1_unit',E_1_unit);
      | set_param([LithiumIonBattery],'E0','E0');
      | set_param([LithiumIonBattery],'E0_unit',E0_unit);
      | set_param([LithiumIonBattery],'E1','E1');
      | set_param([LithiumIonBattery],'E1_unit',E1_unit);
      | set_param([LithiumIonBattery],'E2','E2');
      | set_param([LithiumIonBattery],'E2_unit',E2_unit);
      | set_param([LithiumIonBattery],'E3','E3');
      | set_param([LithiumIonBattery],'E3_unit',E3_unit);
      | set_param([LithiumIonBattery],'Elog','Elog');
      | set_param([LithiumIonBattery],'Elog_unit',Elog_unit);
      | set_param([LithiumIonBattery],'R0','R0');
      | set_param([LithiumIonBattery],'R0_unit',R0_unit);
      | set_param([LithiumIonBattery],'R1','R1');
      | set_param([LithiumIonBattery],'R1_unit',R1_unit);
      | set_param([LithiumIonBattery],'C1','C1');
      | set_param([LithiumIonBattery],'C1_unit',C1_unit);
      | set_param([LithiumIonBattery],'M','M');
      | set_param([LithiumIonBattery],'M_unit',M_unit);
      | set_param([LithiumIonBattery],'alpha','alpha');
      mask Help: eval('open \documentation\lithium_ion_battery_i.pdf')
      mask TypeOptions Q_unit: A*hr
      mask TypeOptions E_1_unit: V
      mask TypeOptions E0_unit: V
      mask TypeOptions E1_unit: V
      mask TypeOptions E2_unit: V
      mask TypeOptions E3_unit: V
      mask TypeOptions Elog_unit: V
      mask TypeOptions R0_unit: Ohm
      mask TypeOptions R1_unit: Ohm
      mask TypeOptions C1_unit: F
      mask TypeOptions M_unit: V
      mask Display:
      | modelname = [gcb];
      | % image(imread("library\+pmsm_dq2\pmsm_drawing_mask.png"));
      | 
      | color('blue')
      | port_label('rconn',1,'Uout+');
      | port_label('rconn',2,'Uout-');
      | color('blue')
      | port_label('lconn',1,'Uin+');
      | port_label('lconn',2,'Uin-');
      | color('black')
      | port_label('output',1,'LithiumIonBattery_Data');
  LithiumIonBattery_Data : Scope  NumInputPorts=2
  PEMFC : Subsystem  mask{Va=4e-6, Va_unit=m^3, Vc=4e-6, Vc_unit=m^3, Ncells=348, Rohm0=0.42, Rohm0_unit=Ohm, Ract=0.42, Ract_unit=Ohm, Rconc=0.42, Rconc_unit=Ohm, Cdlc=2, Cdlc_unit=F}
      mask prompts: Va "Anode Volume"; Vc "Cathode Volume"; Ncells "Number of Cells in Series"; Rohm0 "R ohm0"; Ract "R act"; Rconc "R conc"; Cdlc "Double Layer Capacitance"
      mask init:
      | pemfc_stack = [gcb, '/pemfc_stack'];
      | set_param([pemfc_stack],'Va','Va');
      | set_param([pemfc_stack],'Va_unit',Va_unit);
      | set_param([pemfc_stack],'Vc','Vc');
      | set_param([pemfc_stack],'Vc_unit',Va_unit);
      | set_param([pemfc_stack],'Ncells','Ncells');
      | set_param([pemfc_stack],'Rohm0','Rohm0');
      | set_param([pemfc_stack],'Rohm0_unit',Rohm0_unit);
      | set_param([pemfc_stack],'Ract','Ract');
      | set_param([pemfc_stack],'Ract_unit',Ract_unit);
      | set_param([pemfc_stack],'Rconc','Rconc');
      | set_param([pemfc_stack],'Rconc_unit',Rconc_unit);
      | set_param([pemfc_stack],'Cdlc','Cdlc');
      | set_param([pemfc_stack],'Cdlc_unit',Cdlc_unit);
      mask Help: eval('open \documentation\permfc_simscape_model.pdf')
      mask DialogControl PEMFCStackParameters Prompt: PEM FC Stack Parameters
      mask Display:
      | modelname = [gcb];
      | % image(imread("library\+pmsm_dq2\pmsm_drawing_mask.png"));
      | 
      | color('blue')
      | port_label('rconn',1,'Uout+');
      | color('blue')
      | port_label('rconn',2,'Uout-');
      | color('black')
      | port_label('output',1,'PEMFC_Data');
  PEMFC_Data : Scope
  PMSM_Data : Scope
  Selector : Selector  InputPortWidth=4  IndexOptions=Index vector (dialog)  Indices=[2 1]  OutputSizes=1
  Unit Delay4 : UnitDelay  SampleTime=tsample  HasFrameUpgradeWarning=on
  battery_management : Subsystem
  dc/dc : Subsystem
  pmsm_ctrl : Subsystem
  D : PMIOPort  Side=Right
  wires:
  dc/dc/1(DC/DC_Data) -> DCDC_Data/1
  PEMFC/1(PEMFC_Data) -> PEMFC_Data/1
  pmsm_ctrl/1(PMSM_Data) -> PMSM_Data/1
  Selector/1 -> Demux/1
  Demux/1 -> battery_management/1(vout(k))
  Demux/2 -> battery_management/2(i(k))
  LithiumIonBattery/1(lithiumIonBattery_Data) -> Unit Delay4/1, LithiumIonBattery_Data/1
  battery_management/1(SOC(k)) -> LithiumIonBattery_Data/2
  Unit Delay4/1 -> Selector/1
  connections:
  PEMFC/RConn2 -- dc/dc/LConn2
  pmsm_ctrl/LConn2 -- LithiumIonBattery/RConn2
  dc/dc/RConn2 -- LithiumIonBattery/LConn2
  dc/dc/RConn1 -- LithiumIonBattery/LConn1
  dc/dc/LConn1 -- PEMFC/RConn1
  pmsm_ctrl/LConn1 -- LithiumIonBattery/RConn1
  pmsm_ctrl/RConn1 -- D/RConn1

== system hdv_hydroelectropowertrain_model/PR776_powertrain/front_blade_model ==
  blade_height : Subsystem
  hose : Subsystem
  piston_tilt : Subsystem
  pistons_height : Subsystem
  pistons_pitch : Subsystem
  pitch_load : Subsystem
  tilt_load : Subsystem
  vertical_load : Subsystem
  A : PMIOPort  Side=Left
  B : PMIOPort  Port=2  Side=Left
  wires:
  blade_height/1(blade_height) -> piston_tilt/1(ref), pistons_pitch/1(ref), pistons_height/1(ref)
  connections:
  hose/LConn2 -- B/RConn1
  hose/RConn1 -- piston_tilt/LConn1 -- pistons_pitch/LConn1 -- pistons_height/LConn1
  hose/RConn2 -- piston_tilt/LConn2 -- pistons_pitch/LConn2 -- pistons_height/LConn2
  vertical_load/LConn1 -- pistons_height/RConn1
  hose/LConn1 -- A/RConn1
  piston_tilt/RConn1 -- tilt_load/RConn1
  pitch_load/RConn1 -- pistons_pitch/RConn1

== system hdv_hydroelectropowertrain_model/PR776_powertrain/load_distribution ==
  loadA : Inport
  loadB : Inport  Port=2
  PS Product : fl_lib/Physical Signals/Functions/PS Product
  PS Product1 : fl_lib/Physical Signals/Functions/PS Product
  PS Sign : fl_lib/Physical Signals/Nonlinear Operators/PS Sign
      settings: InternalSimscapePortConfiguration="{\"Bottom\":[],\"Left\":[{\"id\":\"I\",\"label\":\"\",\"type\":\"input\"}],\"Right\":[{\"id\":\"O\",\"label\":\"\",\"type\":\"output\"}],\"Top\":[]}"
  PS Sign1 : fl_lib/Physical Signals/Nonlinear Operators/PS Sign
      settings: InternalSimscapePortConfiguration="{\"Bottom\":[],\"Left\":[{\"id\":\"I\",\"label\":\"\",\"type\":\"input\"}],\"Right\":[{\"id\":\"O\",\"label\":\"\",\"type\":\"output\"}],\"Top\":[]}"
  PS Transfer Function : fl_lib/Physical Signals/Linear Operators/PS Transfer Function  transfer_function_type=foundation.enum.transfer_function_type.lag  T=1 s  T1=2 s  T2=1 s  reset_method=foundation.enum.IntegratorResetSpec.None  initial_condition_spec=foundation.enum.IntegratorICSpec.Internal  y0=0 N*m
      settings: InternalSimscapePortConfiguration="{\"Bottom\":[],\"Left\":[{\"id\":\"U\",\"label\":\"\",\"type\":\"input\"}],\"Right\":[{\"id\":\"Y\",\"label\":\"\",\"type\":\"output\"}],\"Top\":[]}"
  PS Transfer Function1 : fl_lib/Physical Signals/Linear Operators/PS Transfer Function  transfer_function_type=foundation.enum.transfer_function_type.lag  T=1 s  T1=2 s  T2=1 s  reset_method=foundation.enum.IntegratorResetSpec.None  initial_condition_spec=foundation.enum.IntegratorICSpec.Internal  y0=0 N*m
      settings: InternalSimscapePortConfiguration="{\"Bottom\":[],\"Left\":[{\"id\":\"U\",\"label\":\"\",\"type\":\"input\"}],\"Right\":[{\"id\":\"Y\",\"label\":\"\",\"type\":\"output\"}],\"Top\":[]}"
  Simulink-PS Converter5 : nesl_utility/Simulink-PS Converter  PhysicalDomain=network_engine_domain  SubClassName=ps_input  LeftPortType=input  RightPortType=output  PseudoPeriodic=off  Frequencies=[]  NoiseDistribution=none  NoiseParameters=[]  Unit=N*m  AffineConversion=off  FilteringAndDerivatives=provide  SimscapeFilterOrder=1  InputFilterTimeConstant=0.001  UdotUserProvided=0
  Simulink-PS Converter6 : nesl_utility/Simulink-PS Converter  PhysicalDomain=network_engine_domain  SubClassName=ps_input  LeftPortType=input  RightPortType=output  PseudoPeriodic=off  Frequencies=[]  NoiseDistribution=none  NoiseParameters=[]  Unit=N*m  AffineConversion=off  FilteringAndDerivatives=provide  SimscapeFilterOrder=1  InputFilterTimeConstant=0.001  UdotUserProvided=0
  PS Sign2 : PMIOPort  Side=Left
  Load_RD : PMIOPort  Port=2  Side=Right
  PS Sign3 : PMIOPort  Port=3  Side=Left
  Load_LD : PMIOPort  Port=4  Side=Right
  wires:
  loadA/1 -> Simulink-PS Converter5/1
  loadB/1 -> Simulink-PS Converter6/1
  connections:
  PS Product1/RConn1 -- PS Transfer Function/LConn1
  PS Sign1/RConn1 -- PS Product1/LConn1
  PS Product1/LConn2 -- Simulink-PS Converter5/RConn1
  PS Transfer Function/RConn1 -- Load_RD/RConn1
  PS Transfer Function1/RConn1 -- Load_LD/RConn1
  PS Sign/RConn1 -- PS Product/LConn1
  PS Product/RConn1 -- PS Transfer Function1/LConn1
  PS Product/LConn2 -- Simulink-PS Converter6/RConn1
  PS Sign2/RConn1 -- PS Sign1/LConn1
  PS Sign3/RConn1 -- PS Sign/LConn1

== system hdv_hydroelectropowertrain_model/Vehicle Control System/Engine Anti-Stall ==
  1-D Lookup Table : Lookup_n-D  NumberOfTableDimensions=1  BreakpointsForDimension1=rpm_base  Table=available_torque  InternalRulePriority=Speed  RndMeth=Simplest
  Constant1 : Constant  Value=0
  Engine Overload Control : Subsystem  mask{kp=kp_te_comp, ki=ki_te_comp, ts=tsample, sat_pos=1.64, sat_neg=0}
  Engine Torque Compensation : Scope  NumInputPorts=2
  Gain : Gain  Gain=-1
  Sum : Sum  Inputs=|+-
  To Workspace : ToWorkspace  VariableName=engine_compensation  SampleTime=Tc
      settings: MaxDataPoints=Nc
  To Workspace1 : ToWorkspace  VariableName=torque_engine_limit  SampleTime=Tc
      settings: MaxDataPoints=Nc
  Transfer Fcn4 : TransferFcn  Denominator=[1e-4 1]
  tag scope: compensation_engine=global
  wires:
  Transfer Fcn4/1 -> Sum/2
  1-D Lookup Table/1 -> To Workspace1/1, Sum/1
  Engine Overload Control/1(u) -> Gain/1
  [omega_engine_reference] -> 1-D Lookup Table/1
  [tau_e] -> Transfer Fcn4/1
  Constant1/1 -> Engine Overload Control/2(xref)
  Sum/1 -> Engine Torque Compensation/2, Engine Overload Control/1(x)  "tau_e_error"
  Gain/1 -> To Workspace/1, Engine Torque Compensation/1, [compensation_engine]  "engine torque compensation"

== system hdv_hydroelectropowertrain_model/Vehicle Control System/Over Pressure Compensation ==
  Abs : Abs  SaturateOnIntegerOverflow=off
  Abs1 : Abs  SaturateOnIntegerOverflow=off
  Mux2 : Mux  Inputs=2
  Pressure Compensation : Scope  NumInputPorts=2
  Pressure Compensation Control A : Subsystem  mask{kp=kp_dp_comp, ki=ki_dp_comp, ts=tsample, sat_pos=0, sat_neg=-1.64}
  Pressure Compensation Control B : Subsystem  mask{kp=kp_dp_comp, ki=ki_dp_comp, ts=tsample, sat_pos=0, sat_neg=-1.64}
  To Workspace : ToWorkspace  VariableName=dp1_compensation  SampleTime=Tc
      settings: MaxDataPoints=Nc
  To Workspace1 : ToWorkspace  VariableName=dp2_compensation  SampleTime=Tc
      settings: MaxDataPoints=Nc
  Transfer Fcn1 : TransferFcn  Denominator=[1e-4 1]
  Transfer Fcn2 : TransferFcn  Denominator=[1e-4 1]
  direction1 : Subsystem
  direction2 : Subsystem
  dp_max : Constant  Value=dp_lim
  pressure_control_lineA : Scope
  tag scope: compensation_pressureA=global, compensation_pressureB=global
  wires:
  Abs1/1 -> Mux2/1, Pressure Compensation Control A/1(x)  "dpA_measure"
  Transfer Fcn1/1 -> Abs1/1
  [dpBm] -> Transfer Fcn2/1
  dp_max/1 -> Pressure Compensation Control B/2(xref), Pressure Compensation Control A/2(xref), Mux2/2  "dpA_max_ref"
  direction1/1(Out1) -> To Workspace/1, [compensation_pressureA], Pressure Compensation/1  "beta_dpA_compensation"
  Mux2/1 -> pressure_control_lineA/1
  [dpAm] -> Transfer Fcn1/1
  Pressure Compensation Control B/1(u) -> direction2/1(In1)
  direction2/1(Out1) -> To Workspace1/1, [compensation_pressureB], Pressure Compensation/2  "beta_dpB_compensation"
  Transfer Fcn2/1 -> Abs/1
  Pressure Compensation Control A/1(u) -> direction1/1(In1)
  Abs/1 -> Pressure Compensation Control B/1(x)  "dpB_measure"
